simulink model "second_order"  (R2021a)
settings: Solver=VariableStepAuto  StartTime=0.0  StopTime=10.0  MaxStep=0.01  RelTol=1e-3
settings Model: Creator=Beshary  LastModifiedBy=Beshary

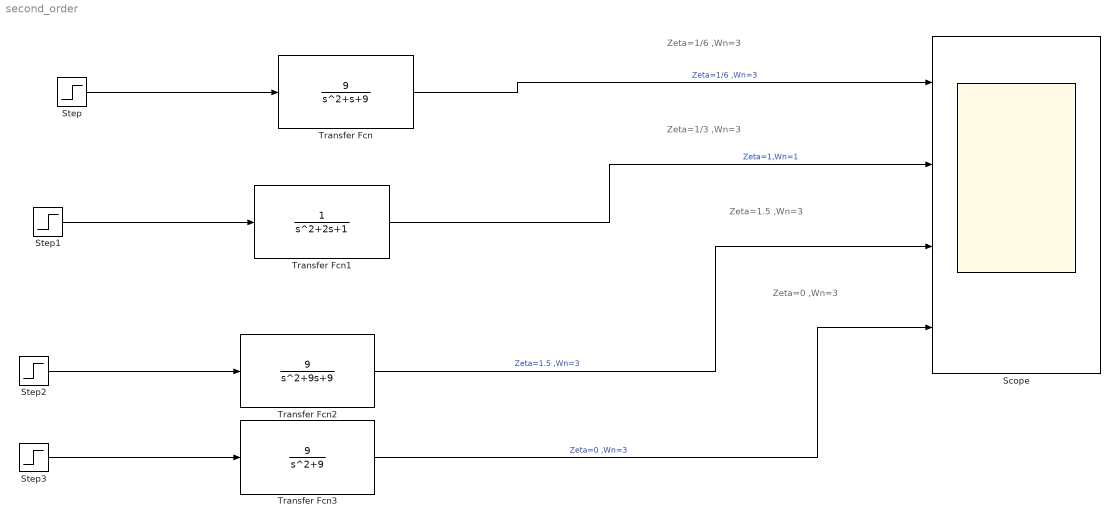
== system second_order ==
  note: Zeta=1/6 ,Wn=3
  note: Zeta=1/3 ,Wn=3
  note: Zeta=1.5 ,Wn=3
  note: Zeta=0 ,Wn=3
  Scope : Scope  NumInputPorts=4
  Step{,1..3} (4 alike) : Step  SampleTime=0
  Transfer Fcn : TransferFcn  Numerator=[9]  Denominator=[1 1 9]
  Transfer Fcn1 : TransferFcn
  Transfer Fcn2 : TransferFcn  Numerator=[9]  Denominator=[1 9 9]
  Transfer Fcn3 : TransferFcn  Numerator=[9]  Denominator="[1  0 9]"
  wires:
  Step/1 -> Transfer Fcn/1
  Transfer Fcn/1 -> Scope/1  "Zeta=1/6 ,Wn=3"
  Transfer Fcn1/1 -> Scope/2  "Zeta=1,Wn=1"
  Step1/1 -> Transfer Fcn1/1
  Step2/1 -> Transfer Fcn2/1
  Transfer Fcn2/1 -> Scope/3  "Zeta=1.5 ,Wn=3"
  Transfer Fcn3/1 -> Scope/4  "Zeta=0 ,Wn=3"
  Step3/1 -> Transfer Fcn3/1
